simulink library "Driver_PI"  (R2018b)
settings: Solver=VariableStepAuto  StartTime=0.0  StopTime=10.0  RelTol=1e-3
undefined symbols (not defined in the file): magnitude
libraries: simulink x2
settings Model: Creator=ga69qig  LastModifiedBy=ga69qig
settings SFSimCC: SimUseLocalCustomCode=off
settings RTWCC: RTWUseLocalCustomCode=off

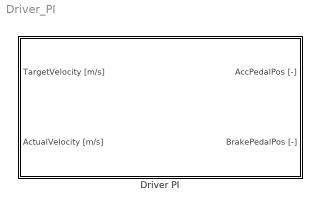
== system Driver_PI ==
  Driver PI : Subsystem  mask(SB){ThrottleP=14, ThrottleI=0.12, BrakeP=14, BrakeI=0.12, WeightingFactorPrecontrol=0, MaxVehicleSpeed=80, hysteresis=0.2, LocalSampleTime=-1}
      mask prompts: ThrottleP "Throttle P-Value [-]"; ThrottleI "Throttle I-Value [-]"; BrakeP "Brake P-Value [-]"; BrakeI "Brake I-Value [-]"; WeightingFactorPrecontrol "Weighting Factor Precontrol [-]"; MaxVehicleSpeed "Maximum Vehicle Speed [m/s]"; hysteresis "Hysteresis Corridor [m/s]"; LocalSampleTime "Local System Sample-Time [s]"
      mask help:
      | <Author> Alexander Koch, Benedikt Danquah based on Stefan Müller [1], Stephan Rohr [2]  </Author>
      | <Date> 02/11/2018 </Date>
      |
      | <Description>
      | A Longitudinal controller containing one PI-Controller for acceleration and one PI-controller for braking is included. The block creates an acceleration pedal position between 0 and 1 and a braking peadal position between 0 and 1. Based on the velocity deviation a hysteresis control decides which controler is activated. A precontrol adds acceleration pedal value based on the target velocity. The value is normalized by the maximum velocity of the vehicle.
      | </Description>
      mask init:
      | GlobalSampleTime = CalcGlobalSampleTime(LocalSampleTime);
      mask Help:
      | <Parameters>
      | Throttle P-Value [-]
      | Throttle I-Value [-]
      | Brake P-Value [-]
      | Brake I-Value [-]
      | Weighting Factor Precontrol [-]
      | Maximum Vehicle Speed [m/s]
      | Value hysteresis Corridor [m/s]
      | Local System Sample-Time [s]
      | 	<Min> GlobalSampleTime </Min>
      | Global Sample-Time [s]
      | </Parameters>
      | 
      | <Inputs>
      | TargetVelocity [m/s]
      | ActualVelocity [m/s]
      | </Inputs>
      | 
      | <Outputs>
      | AccPedalPos [-]
      | 	<Min> 0 </Min>
      | 	<Max> 1 </Max>
      | BrakePedalPos [-]
      | 	<Min> 0 </Min>
      | 	<Max> 1 </Max>
      | </Outputs>
      | 
      | <Sources>
      | [1] S. Mueller, S. Rohr, W. Schmid, and M. Lienkamp, “Analysing the Influence of Driver Behaviour and Tuning Measures on Battery Aging and Residual Value of Electric Vehicles,” in Proc. EVS30 Symposium, Stuttgart, 2017, pp. 1–12.
      | [2] S. Rohr, “Technisch-wirtschaftliche Analyse des Zweitnutzungs- potentials von Lithium-Ionen-Traktionsbatterien,” Dissertation, Institute of Automotive Technology, Technical University Munich, Munich, 2018.
      | </Sources>
      mask TypeOptions LocalSampleTime: TargetVelocity [m//s]/SampleTime | ActualVelocity [m//s]/SampleTime
      mask DialogControl Container3 Prompt: Documentation:
      mask DialogControl DescHelpVar Prompt: %<MaskHelp>
      mask DialogControl Container5 Prompt: Throttle
      mask DialogControl Container6 Prompt: Break
      mask DialogControl Container7 Prompt: Precontrol
      mask DialogControl Container8 Prompt: Sample Time
      mask Display:
      | [picturexpos,pictureypos,picturewidth,pictureheight] = ...
      |     CalcBlockPicturePosition(gcb,1,0.01,0.1,80,80); % calculating picture position depending on Block size and minimum margin size
      | image('Driver_PI.svg',[picturexpos pictureypos picturewidth pictureheight]) % plot picture to block

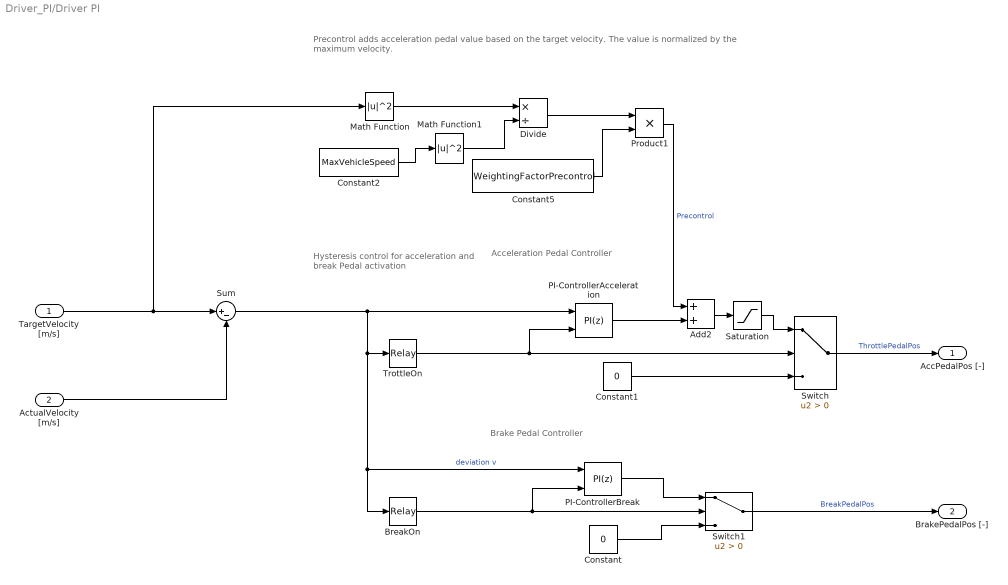
== system Driver_PI/Driver PI ==
  note: Precontrol adds acceleration pedal value
      | based on the target velocity. The value is
      | normalized by the maximum velocity.
  note: Acceleration Pedal Controller
  note: Brake Pedal Controller
  note: Hysteresis control for
      | acceleration and break
      | Pedal activation
  TargetVelocity [m/s] : Inport  SampleTime=LocalSampleTime
  ActualVelocity [m/s] : Inport  Port=2  SampleTime=LocalSampleTime
  Add2 : Sum
  BreakOn : Relay  OnSwitchValue=hysteresis  OffSwitchValue=-hysteresis  OnOutputValue=0  OffOutputValue=1
  Constant : Constant  Value=0
  Constant1 : Constant  Value=0
  Constant2 : Constant  Value=MaxVehicleSpeed
  Constant5 : Constant  Value=WeightingFactorPrecontrol
  Divide : Product  Inputs=*/
  Math Function : Math  Operator=magnitude^2  SaturateOnIntegerOverflow=on
  Math Function1 : Math  Operator=magnitude^2  SaturateOnIntegerOverflow=on
  PI-ControllerAcceleration : simulink/Continuous/PID Controller  Controller=PI  Form=Parallel  TimeDomain=Discrete-time  SampleTime=-1  IntegratorMethod=Forward Euler  FilterMethod=Forward Euler  ControllerParametersSource=internal  P=ThrottleP  I=ThrottleI  D=0  UseFilter=on  N=100  TunerSelectOption=Transfer Function Based (PID Tuner App)  InitialConditionSource=internal  InitialConditionForIntegrator=0  InitialConditionForFilter=0  DifferentiatorICPrevScaledInput=0  ExternalReset=rising  TrackingMode=off  Kt=1  LimitOutput=on  UpperSaturationLimit=1  LowerSaturationLimit=0  LinearizeAsGain=off  AntiWindupMode=none  Kb=1  POutMin=[]  POutMax=[]  IOutMin=[]  IOutMax=[]  DOutMin=[]  DOutMax=[]  NOutMin=[]  NOutMax=[]  SumOutMin=[]  SumOutMax=[]  SaturationOutMin=[]  SaturationOutMax=[]  PParamMin=[]  PParamMax=[]  IParamMin=[]  IParamMax=[]  DParamMin=[]  DParamMax=[]  NParamMin=[]  NParamMax=[]  KbParamMin=[]  KbParamMax=[]  KtParamMin=[]  KtParamMax=[]  KbOutMin=[]  KbOutMax=[]  KtOutMin=[]  KtOutMax=[]  IntegratorOutMin=[]  IntegratorOutMax=[]  FilterOutMin=[]  FilterOutMax=[]  SumI1OutMin=[]  SumI1OutMax=[]  SumI2OutMin=[]  SumI2OutMax=[]  SumI3OutMin=[]  SumI3OutMax=[]  SumI4OutMin=[]  SumI4OutMax=[]  SumDOutMin=[]  SumDOutMax=[]  DifferentiatorOutMin=[]  DifferentiatorOutMax=[]  FilterDiffOutCoefMin=[]  FilterDiffOutCoefMax=[]  ReciprocalOutMin=[]  ReciprocalOutMax=[]  SumDenOutMin=[]  SumDenOutMax=[]  SumNumOutMin=[]  SumNumOutMax=[]  DivideOutMin=[]  DivideOutMax=[]  IntegratorContinuousStateAttributes=''  IntegratorStateMustResolveToSignalObject=off  IntegratorRTWStateStorageClass=Auto  FilterContinuousStateAttributes=''  FilterStateMustResolveToSignalObject=off  FilterRTWStateStorageClass=Auto  ParallelPVariant=InternalParameters  IdealPVariant=Disabled  IVariant=InternalParameters  DVariant=Disabled  IntegratorVariant=Discrete  SatVariant=Enabled  AWVariant=Passthrough  PCopyVariant=Disabled  TRVariant=Disabled  FdbkBlocksVariant=Forward  IdealPFdbkVariant=Disabled  SatFdbkVariant=Disabled  DerivativeFilterVariant=Disabled  NVariant=Disabled  NCopyVariant=Disabled_SignalSpec  FilterICVariant=Disabled  IntegratorICVariant=InternalICs  ExternalResetVariant=ExternalReset  TRSumVariant=Passthrough  SumFdbkVariant=Disabled  SumVariant=Sum_PI
  PI-ControllerBreak : simulink/Continuous/PID Controller  Controller=PI  Form=Parallel  TimeDomain=Discrete-time  SampleTime=-1  IntegratorMethod=Forward Euler  FilterMethod=Forward Euler  ControllerParametersSource=internal  P=-BrakeP  I=-BrakeI  D=0  UseFilter=on  N=100  TunerSelectOption=Transfer Function Based (PID Tuner App)  InitialConditionSource=internal  InitialConditionForIntegrator=0  InitialConditionForFilter=0  DifferentiatorICPrevScaledInput=0  ExternalReset=rising  TrackingMode=off  Kt=1  LimitOutput=on  UpperSaturationLimit=1  LowerSaturationLimit=0  LinearizeAsGain=off  AntiWindupMode=none  Kb=1  POutMin=[]  POutMax=[]  IOutMin=[]  IOutMax=[]  DOutMin=[]  DOutMax=[]  NOutMin=[]  NOutMax=[]  SumOutMin=[]  SumOutMax=[]  SaturationOutMin=[]  SaturationOutMax=[]  PParamMin=[]  PParamMax=[]  IParamMin=[]  IParamMax=[]  DParamMin=[]  DParamMax=[]  NParamMin=[]  NParamMax=[]  KbParamMin=[]  KbParamMax=[]  KtParamMin=[]  KtParamMax=[]  KbOutMin=[]  KbOutMax=[]  KtOutMin=[]  KtOutMax=[]  IntegratorOutMin=[]  IntegratorOutMax=[]  FilterOutMin=[]  FilterOutMax=[]  SumI1OutMin=[]  SumI1OutMax=[]  SumI2OutMin=[]  SumI2OutMax=[]  SumI3OutMin=[]  SumI3OutMax=[]  SumI4OutMin=[]  SumI4OutMax=[]  SumDOutMin=[]  SumDOutMax=[]  DifferentiatorOutMin=[]  DifferentiatorOutMax=[]  FilterDiffOutCoefMin=[]  FilterDiffOutCoefMax=[]  ReciprocalOutMin=[]  ReciprocalOutMax=[]  SumDenOutMin=[]  SumDenOutMax=[]  SumNumOutMin=[]  SumNumOutMax=[]  DivideOutMin=[]  DivideOutMax=[]  IntegratorContinuousStateAttributes=''  IntegratorStateMustResolveToSignalObject=off  IntegratorRTWStateStorageClass=Auto  FilterContinuousStateAttributes=''  FilterStateMustResolveToSignalObject=off  FilterRTWStateStorageClass=Auto  ParallelPVariant=InternalParameters  IdealPVariant=Disabled  IVariant=InternalParameters  DVariant=Disabled  IntegratorVariant=Discrete  SatVariant=Enabled  AWVariant=Passthrough  PCopyVariant=Disabled  TRVariant=Disabled  FdbkBlocksVariant=Forward  IdealPFdbkVariant=Disabled  SatFdbkVariant=Disabled  DerivativeFilterVariant=Disabled  NVariant=Disabled  NCopyVariant=Disabled_SignalSpec  FilterICVariant=Disabled  IntegratorICVariant=InternalICs  ExternalResetVariant=ExternalReset  TRSumVariant=Passthrough  SumFdbkVariant=Disabled  SumVariant=Sum_PI
  Product1 : Product
  Saturation : Saturate  UpperLimit=1  LowerLimit=0
  Sum : Sum  Inputs=|+-
  Switch : Switch  Criteria=u2 > Threshold
  Switch1 : Switch  Criteria=u2 > Threshold
  TrottleOn : Relay  OnSwitchValue=hysteresis  OffSwitchValue=-hysteresis
  AccPedalPos [-] : Outport  SampleTime=GlobalSampleTime
  BrakePedalPos [-] : Outport  Port=2  SampleTime=GlobalSampleTime
  wires:
  Saturation/1 -> Switch/1
  Add2/1 -> Saturation/1
  Math Function/1 -> Divide/1
  Constant2/1 -> Math Function1/1
  Product1/1 -> Add2/1  "Precontrol"
  Math Function1/1 -> Divide/2
  Constant5/1 -> Product1/2
  Divide/1 -> Product1/1
  TrottleOn/1 -> Switch/2, PI-ControllerAcceleration/2
  PI-ControllerBreak/1 -> Switch1/1
  Constant1/1 -> Switch/3
  Constant/1 -> Switch1/3
  Switch/1 -> AccPedalPos [-]/1  "ThrottlePedalPos"
  PI-ControllerAcceleration/1 -> Add2/2
  BreakOn/1 -> Switch1/2, PI-ControllerBreak/2
  ActualVelocity [m/s]/1 -> Sum/2
  Switch1/1 -> BrakePedalPos [-]/1  "BreakPedalPos"
  Sum/1 -> PI-ControllerAcceleration/1, TrottleOn/1, PI-ControllerBreak/1, BreakOn/1  "deviation v"
  TargetVelocity [m/s]/1 -> Sum/1, Math Function/1
